simulink model "WK_MaoBi_Record"  (Simulink 7.7)
settings: Solver=ode4  StartTime=0.0  StopTime=inf  FixedStep=sample_time  RelTol=1e-3
InitFcn:
  | sample_time=0.005;%0.004;%0.0025;%0.02;
  | DeltaT = 0.02;
  | g = 9.81;
  | H0 = g%0.3165;
  | Kl = 1;
  | 
  | Omega_r = 1.6;%for Horizontal reference
  | Zeta_r = 0.7; %for Horizontal reference
  | Omega = 1.8;%for Horizontal Control
  | Zeta = 0.5;    %for Horizontal Control
  | 
  | Omega_h_r = 2.5; %for vertical reference
  | Zeta_h_r = 0.8;  %for vertical reference
  | Omega_h = 2.7;    %for vertical control
  | Zeta_h = 0.8;         %for vertical control
  | PI=pi;
  | 
  | Mass = 1;
  | Acc_Max = 4;
  | Acc_Max_h = 4;
  | 
  | Max_RP = 60;
undefined symbols (not defined in the file or in its folder): DiscIntNeverNeededParam
libraries: simulink x7, dspadpt3 x3, X330_Control x2, X400_Control x1
(part 1 of 2)
settings Model: Creator=ttcl3  LastModifiedBy=Vicon
settings SolverCC: MaxConsecutiveMinStep=auto
settings DebuggingCC: MultiTaskRateTransMsg=warning
settings SFSimCC: SimParseCustomCode=off

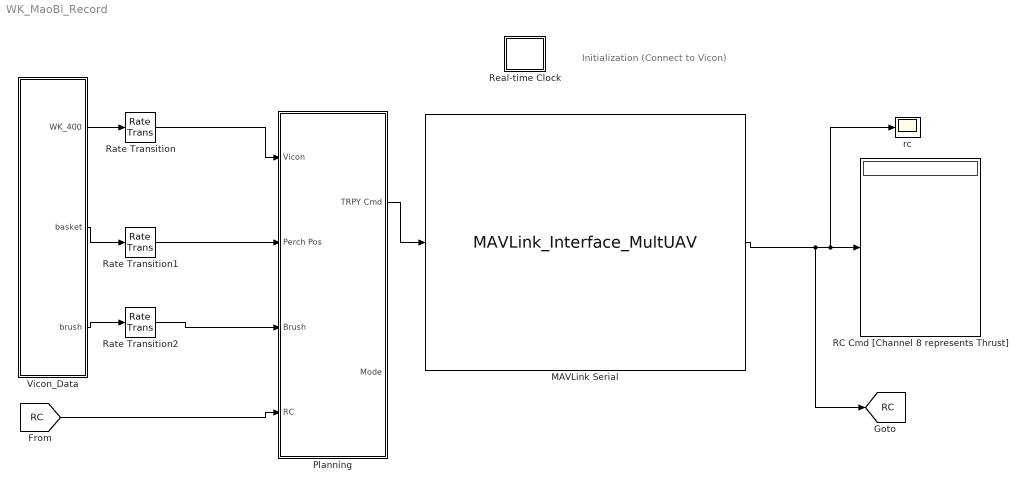
== system WK_MaoBi_Record ==
  note: Initialization
      | (Connect to Vicon)
  MAVLink Serial : S-Function  FunctionName=MAVLink_Interface_MultUAV  Parameters=COM_Port,Baud_Rate,MSG_INPUT,MSG_OUTPUT  EnableBusSupport=off  mask{COM_Port='COM8', Baud_Rate=57600, RC_SCALED=on, Quad_1=on, Quad_2=off, Quad_3=off}
      mask prompts: COM_Port "COM Port"; Baud_Rate "Baud Rate"; RC_SCALED "RC CHANNELS SCALED"; Quad_1 "Quad No 1"; Quad_2 "Quad No 2"; Quad_3 "Quad No 3"
      mask init:
      | MSG_ID_NUM_INPUT = [uint8(196) uint8(197) uint8(198)];
      | MSG_ID_NAME_INPUT = [Quad_1 Quad_2 Quad_3];
      | 
      | MSG_ID_NUM_OUTPUT = [uint8(34)];
      | MSG_ID_NAME_OUTPUT = [RC_SCALED];
      | 
      | idx_input = find(MSG_ID_NAME_INPUT);
      | MSG_INPUT = MSG_ID_NUM_INPUT(idx_input);
      | 
      | idx_output = find(MSG_ID_NAME_OUTPUT);
      | MSG_OUTPUT = MSG_ID_NUM_OUTPUT(idx_output);
      mask TabNameString: Setting,Setting,Output Message,Input Message,Input Message,Input Message
      mask Display:
      | % Block image
      | image(imread('10-inch Quad Heat Map.png'));
      | 
      | %Label block
      | fprintf('MAVLink Serial\n%s\n%dbps', COM_Port,  Baud_Rate)
      | 
      | 
      | %Label input ports
      | 
      | in = 1;
      | if (Quad_1 == 1)
      |     port_label('input', in, 'Quad 1');
      |     in = in + 1;
      | end
      | if (Quad_2 == 1)
      |     port_label('input', in, 'Quad 2');
      |     in = in + 1;
      | end
      | 
      | if (Quad_3 == 1)
      |     port_label('input', in, 'Quad 3');
      |     in = in + 1;
      | end
      | 
      | %Label output ports
      | 
      | out = 1;
      | if (RC_SCALED == 1)
      |     port_label('output', out, 'RC CMD');
      |     out = out + 1;
      | end
  Planning : Subsystem
  RC Cmd [Channel 8 represents Thrust] : Display
  Rate Transition : RateTransition  OutPortSampleTime=0.02
  Rate Transition1 : RateTransition  OutPortSampleTime=0.02
  Rate Transition2 : RateTransition  OutPortSampleTime=0.02
  Real-time Clock : Subsystem  mask(Real-time Clock){sample_time=0.02, tolerance=1}
      mask prompts: sample_time "Synchronize with real-time every n seconds:"; tolerance "Real-time warning tolerance (seconds):"
      mask help: Real-time Synchronization Block
      mask Help: This block synchronizes simulation time with the PC real-time clock or UNIX system clock. The first dialog entry is the period at which the clock is checked to insure real-time synchronization. The second dialog entry is the number of seconds that the simulation time must be within real-time before a warning is printed.
      mask Display: plot(0,0,100,100,[40,60,60,54,54,64,69,76,82,77,81,83,83,81,78,74,70,64,57,49,41,35,32,30,30,31,34,40,47,47,40,40],[90,90,85,85,80,79,76,87,80,70,64,57,49,41,33,28,24,22,21,23,25,31,37,46,56,65,73,78,80,85,85,90],[69,53,53],[64,50,73])
  Vicon_Data : Subsystem
  rc : Scope
      settings: TimeRange=10  YMin=-1  YMax=0.1
  tag scope: RC=global
  wires:
  [RC] -> Planning/4(RC)
  Planning/1(TRPY Cmd) -> MAVLink Serial/1
  MAVLink Serial/1 -> [RC], RC Cmd [Channel 8 represents Thrust]/1, rc/1
  Vicon_Data/1(WK_400) -> Rate Transition/1
  Vicon_Data/2(basket) -> Rate Transition1/1
  Rate Transition/1 -> Planning/1(Vicon)
  Rate Transition1/1 -> Planning/2(Perch Pos)
  Vicon_Data/3(brush) -> Rate Transition2/1
  Rate Transition2/1 -> Planning/3(Brush)

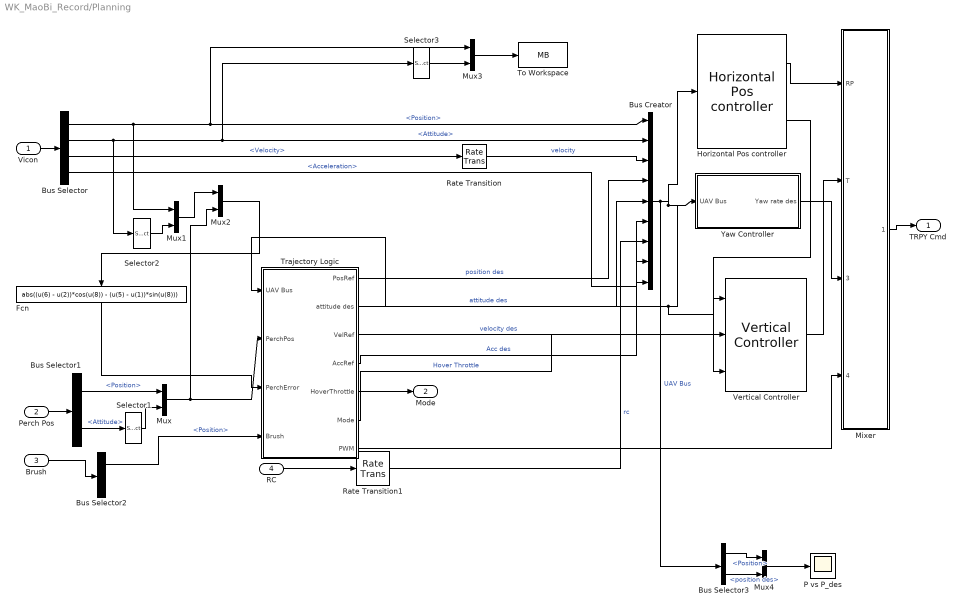
== system WK_MaoBi_Record/Planning ==
  Vicon : Inport
  Perch Pos : Inport  Port=2
  Brush : Inport  Port=3
  RC : Inport  Port=4
  Bus Creator : BusCreator  Inputs=9
  Bus Selector : BusSelector  OutputSignals=Position,Attitude,Velocity,Acceleration
  Bus Selector1 : BusSelector  OutputSignals=Position,Attitude
  Bus Selector2 : BusSelector  OutputSignals=Position,Attitude
  Bus Selector3 : BusSelector  OutputSignals=Position,position des
  Fcn : Fcn  Expr=abs((u(6) - u(2))*cos(u(8)) - (u(5) - u(1))*sin(u(8)))
  Horizontal Pos controller : X330_Control/Horizontal Pos controller  SystemSampleTime=-1  Max_RP=Max_RP  Omega=Omega  PID_i=1  Zeta=Zeta
  Mixer : Subsystem
  Mux{,1..4} (5 alike) : Mux  Inputs=2
  P vs P_des : Scope
      settings: YMin=-1.1  YMax=0.5
  Rate Transition : RateTransition  OutPortSampleTime=0.02
  Rate Transition1 : RateTransition  OutPortSampleTime=0.02
  Selector1 : Selector  InputPortWidth=3  IndexOptions=Index vector (dialog)  Indices=[3]  OutputSizes=1
  Selector2 : Selector  InputPortWidth=3  IndexOptions=Index vector (dialog)  Indices=[3]  OutputSizes=1
  Selector3 : Selector  InputPortWidth=3  IndexOptions=Index vector (dialog)  Indices=[3]  OutputSizes=1
  To Workspace : ToWorkspace  VariableName=MB  SampleTime=0.02  SaveFormat=Structure With Time
  Trajectory Logic : Subsystem
  Vertical Controller : X400_Control/Vertical Controller  SystemSampleTime=-1  Omega_h=Omega_h  Zeta_h=Zeta_h  PID_I_h=1  mass=Mass
  Yaw Controller : Subsystem
  TRPY Cmd : Outport
  Mode : Outport  Port=2
  wires:
  Horizontal Pos controller/1 -> Mixer/1(RP)
  Rate Transition/1 -> Bus Creator/3  "velocity"
  Rate Transition1/1 -> Bus Creator/7  "rc"
  Bus Creator/1 -> Yaw Controller/1(UAV Bus), Trajectory Logic/1(UAV Bus), Vertical Controller/1, Horizontal Pos controller/1, Bus Selector3/1  "UAV Bus"
  Yaw Controller/1(Yaw rate des) -> Mixer/3(Yaw rate)
  Vertical Controller/1 -> Mixer/2(T)
  Bus Selector/4 -> Bus Creator/8  "<Acceleration>"
  Trajectory Logic/1(PosRef) -> Bus Creator/4  "position des"
  Trajectory Logic/2(attitude des) -> Bus Creator/5  "attitude des"
  Trajectory Logic/3(VelRef) -> Bus Creator/6  "velocity des"
  Trajectory Logic/5(HoverThrottle) -> Vertical Controller/2  "Hover Throttle"
  Bus Selector/1 -> Mux1/1, Bus Creator/1, Mux3/1  "<Position>"
  Bus Selector/2 -> Selector2/1, Bus Creator/2, Selector3/1  "<Attitude>"
  Bus Selector/3 -> Rate Transition/1  "<Velocity>"
  Vicon/1 -> Bus Selector/1
  Mixer/1(XYZ RPY) -> TRPY Cmd/1
  Trajectory Logic/4(AccRef) -> Bus Creator/9  "Acc des"
  Mux/1 -> Trajectory Logic/2(PerchPos), Mux2/2
  Trajectory Logic/6(Mode) -> Mode/1
  RC/1 -> Rate Transition1/1
  Trajectory Logic/7(PWM) -> Mixer/4(PWM)
  Perch Pos/1 -> Bus Selector1/1
  Bus Selector1/1 -> Mux/1  "<Position>"
  Bus Selector1/2 -> Selector1/1  "<Attitude>"
  Selector1/1 -> Mux/2
  Selector2/1 -> Mux1/2
  Mux2/1 -> Fcn/1
  Mux1/1 -> Mux2/1
  Fcn/1 -> Trajectory Logic/3(PerchError)
  Horizontal Pos controller/2 -> Vertical Controller/3
  Brush/1 -> Bus Selector2/1
  Bus Selector2/1 -> Trajectory Logic/4(Brush)  "<Position>"
  Mux3/1 -> To Workspace/1
  Selector3/1 -> Mux3/2
  Mux4/1 -> P vs P_des/1
  Bus Selector3/1 -> Mux4/1  "<Position>"
  Bus Selector3/2 -> Mux4/2  "<position des>"

== system WK_MaoBi_Record/Real-time Clock ==
  Real-time Clock : S-Function  FunctionName=rtclock  Parameters=sample_time, tolerance  EnableBusSupport=off

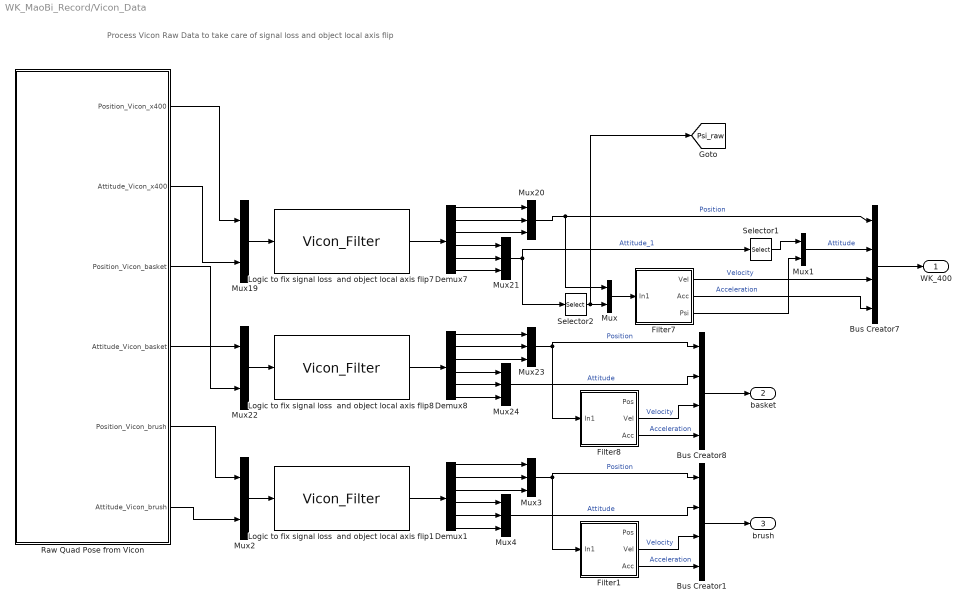
== system WK_MaoBi_Record/Vicon_Data ==
  note: Process Vicon Raw Data to take care of signal loss and object local axis flip
  Bus Creator1 : BusCreator
  Bus Creator7 : BusCreator
  Bus Creator8 : BusCreator
  Demux1 : Demux  Outputs=6
  Demux7 : Demux  Outputs=6
  Demux8 : Demux  Outputs=6
  Filter1 : Subsystem
  Filter7 : Subsystem
  Filter8 : Subsystem
  Logic to fix signal loss  and object local axis flip1 : M-S-Function  FunctionName=Vicon_Filter
  Logic to fix signal loss  and object local axis flip7 : M-S-Function  FunctionName=Vicon_Filter
  Logic to fix signal loss  and object local axis flip8 : M-S-Function  FunctionName=Vicon_Filter
  Mux{,1..2,19,22} (5 alike) : Mux  Inputs=2
  Mux{3..4,20..21,23..24} (6 alike) : Mux  Inputs=3
  Raw Quad Pose from Vicon : Subsystem
  Selector1 : Selector  InputPortWidth=3  IndexOptions=Index vector (dialog)  Indices=[1 2]  OutputSizes=1
  Selector2 : Selector  InputPortWidth=3  IndexOptions=Index vector (dialog)  Indices=[3]  OutputSizes=1
  WK_400 : Outport
  basket : Outport  Port=2
  brush : Outport  Port=3
  tag scope: Psi_raw=global
  wires:
  Mux19/1 -> Logic to fix signal loss  and object local axis flip7/1
  Logic to fix signal loss  and object local axis flip7/1 -> Demux7/1
  Demux7/3 -> Mux20/3
  Demux7/4 -> Mux21/1
  Demux7/5 -> Mux21/2
  Demux7/6 -> Mux21/3
  Bus Creator7/1 -> WK_400/1
  Demux7/1 -> Mux20/1
  Demux7/2 -> Mux20/2
  Mux20/1 -> Bus Creator7/1, Mux/1  "Position"
  Mux22/1 -> Logic to fix signal loss  and object local axis flip8/1
  Logic to fix signal loss  and object local axis flip8/1 -> Demux8/1
  Demux8/3 -> Mux23/3
  Demux8/4 -> Mux24/1
  Demux8/5 -> Mux24/2
  Demux8/6 -> Mux24/3
  Filter8/2(Vel) -> Bus Creator8/3  "Velocity"
  Filter8/3(Acc) -> Bus Creator8/4  "Acceleration"
  Mux24/1 -> Bus Creator8/2  "Attitude"
  Bus Creator8/1 -> basket/1
  Demux8/1 -> Mux23/1
  Demux8/2 -> Mux23/2
  Mux23/1 -> Filter8/1(In1), Bus Creator8/1  "Position"
  Raw Quad Pose from Vicon/1(Position_Vicon_x400) -> Mux19/1
  Raw Quad Pose from Vicon/2(Attitude_Vicon_x400) -> Mux19/2
  Raw Quad Pose from Vicon/3(Position_Vicon_basket) -> Mux22/1
  Raw Quad Pose from Vicon/4(Attitude_Vicon_basket) -> Mux22/2
  Mux21/1 -> Selector2/1, Selector1/1  "Attitude_1"
  Filter7/1(Vel) -> Bus Creator7/3  "Velocity"
  Filter7/2(Acc) -> Bus Creator7/4  "Acceleration"
  Selector2/1 -> Mux/2, [Psi_raw]
  Mux/1 -> Filter7/1(In1)
  Filter7/3(Psi) -> Mux1/2
  Selector1/1 -> Mux1/1
  Mux1/1 -> Bus Creator7/2  "Attitude"
  Mux2/1 -> Logic to fix signal loss  and object local axis flip1/1
  Logic to fix signal loss  and object local axis flip1/1 -> Demux1/1
  Demux1/3 -> Mux3/3
  Demux1/4 -> Mux4/1
  Demux1/5 -> Mux4/2
  Demux1/6 -> Mux4/3
  Filter1/2(Vel) -> Bus Creator1/3  "Velocity"
  Filter1/3(Acc) -> Bus Creator1/4  "Acceleration"
  Mux4/1 -> Bus Creator1/2  "Attitude"
  Bus Creator1/1 -> brush/1
  Demux1/1 -> Mux3/1
  Demux1/2 -> Mux3/2
  Mux3/1 -> Bus Creator1/1, Filter1/1(In1)  "Position"
  Raw Quad Pose from Vicon/5(Position_Vicon_brush) -> Mux2/1
  Raw Quad Pose from Vicon/6(Attitude_Vicon_brush) -> Mux2/2

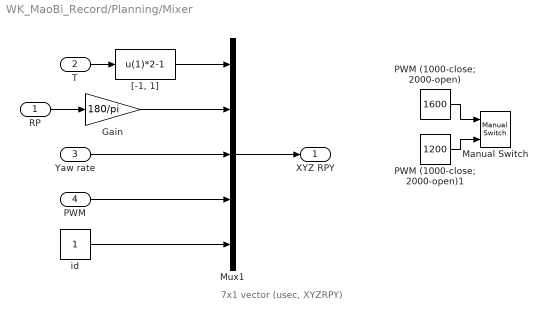
== system WK_MaoBi_Record/Planning/Mixer ==
  note: 7x1 vector (usec, XYZRPY)
  RP : Inport
  T : Inport  Port=2
  Yaw rate : Inport  Port=3
  PWM : Inport  Port=4
  Gain : Gain  Gain=180/pi
  Manual Switch : simulink/Signal Routing/Manual Switch  SystemSampleTime=-1  sw=1  action=0  varsize=off
  Mux1 : Mux  Inputs=5
  PWM (1000-close; 2000-open) : Constant  Value=1600  SampleTime=0.02
  PWM (1000-close; 2000-open)1 : Constant  Value=1200  SampleTime=0.02
  "[-1, 1]" : Fcn  Expr=u(1)*2-1
  id : Constant  SampleTime=0.02
  XYZ RPY : Outport
  wires:
  Mux1/1 -> XYZ RPY/1
  T/1 -> "[-1, 1]"/1
  RP/1 -> Gain/1
  Yaw rate/1 -> Mux1/3
  id/1 -> Mux1/5
  PWM (1000-close; 2000-open)/1 -> Manual Switch/1
  PWM (1000-close; 2000-open)1/1 -> Manual Switch/2
  PWM/1 -> Mux1/4
  Gain/1 -> Mux1/2
  "[-1, 1]"/1 -> Mux1/1

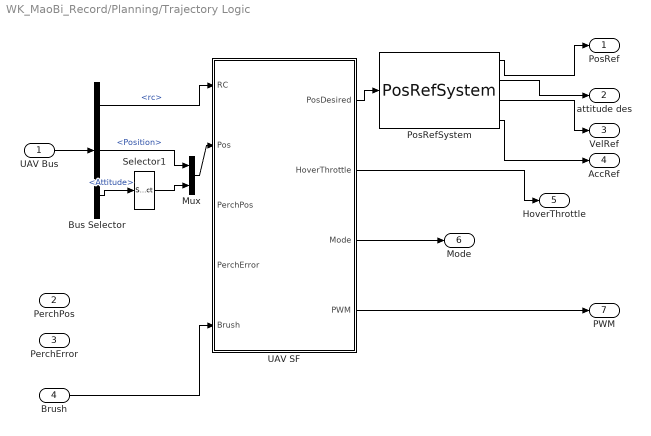
== system WK_MaoBi_Record/Planning/Trajectory Logic ==
  UAV Bus : Inport
  PerchPos : Inport  Port=2
  PerchError : Inport  Port=3
  Brush : Inport  Port=4
  Bus Selector : BusSelector  OutputSignals=rc,Position,Attitude
  Mux : Mux  Inputs=2
  PosRefSystem : X330_Control/PosRefSystem  SystemSampleTime=-1  Omega_r=Omega_r  Zeta_r=Zeta_r  Acc_Max=Acc_Max  Omega_h_r=Omega_h_r  Zeta_h_r=Zeta_h_r  Acc_h_Max=Acc_Max_h
  Selector1 : Selector  InputPortWidth=3  IndexOptions=Index vector (dialog)  Indices=[3]  OutputSizes=1
  UAV SF : Stateflow chart  TreatAsAtomicUnit=on
  PosRef : Outport
  attitude des : Outport  Port=2
  VelRef : Outport  Port=3
  AccRef : Outport  Port=4
  HoverThrottle : Outport  Port=5
  Mode : Outport  Port=6
  PWM : Outport  Port=7
  wires:
  UAV SF/1(PosDesired) -> PosRefSystem/1
  Bus Selector/1 -> UAV SF/1(RC)  "<rc>"
  UAV SF/2(HoverThrottle) -> HoverThrottle/1
  UAV SF/3(Mode) -> Mode/1
  UAV Bus/1 -> Bus Selector/1
  Bus Selector/2 -> Mux/1  "<Position>"
  Bus Selector/3 -> Selector1/1  "<Attitude>"
  Selector1/1 -> Mux/2
  Mux/1 -> UAV SF/2(Pos)
  UAV SF/4(PWM) -> PWM/1
  PosRefSystem/1 -> PosRef/1
  PosRefSystem/3 -> VelRef/1
  PosRefSystem/4 -> AccRef/1
  PosRefSystem/2 -> attitude des/1
  Brush/1 -> UAV SF/5(Brush)

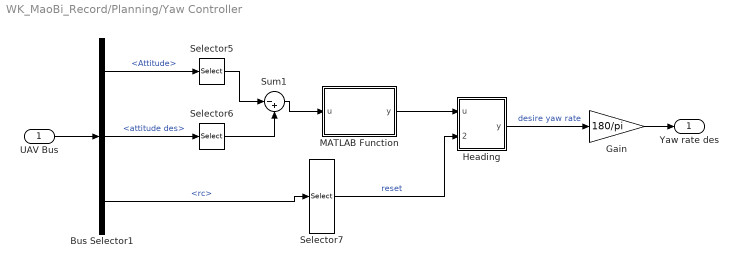
== system WK_MaoBi_Record/Planning/Yaw Controller ==
  UAV Bus : Inport
  Bus Selector1 : BusSelector  OutputSignals=Attitude,attitude des,rc
  Gain : Gain  Gain=180/pi
  Heading : Subsystem  AncestorBlock=simulink/Continuous/PID Controller  DialogController=pidpack.PIDConfig.pidDDGCreate  DialogControllerArgs=DataTag0  mask(PID 1dof){Controller=PI, TimeDomain=Discrete-time, SampleTime=0.02, IntegratorMethod=Trapezoidal, FilterMethod=Trapezoidal, Form=Parallel, P=3, I=1, D=0, N=100, InitialConditionSource=internal, InitialConditionForIntegrator=0, InitialConditionForFilter=0, ExternalReset=rising, IgnoreLimit=off, ZeroCross=on, LimitOutput=on, UpperSaturationLimit=300*pi/180, LowerSaturationLimit=-300*pi/180, LinearizeAsGain=off, AntiWindupMode=none, Kb=1, TrackingMode=off, Kt=1, RndMeth=Floor, SaturateOnIntegerOverflow=off, LockScale=off, PParamMin=[], PParamMax=[], PParamDataTypeStr=Inherit: Inherit via internal rule, IParamMin=[], IParamMax=[], IParamDataTypeStr=Inherit: Inherit via internal rule, DParamMin=[], DParamMax=[], DParamDataTypeStr=Inherit: Inherit via internal rule, NParamMin=[], NParamMax=[], NParamDataTypeStr=Inherit: Inherit via internal rule, KbParamMin=[], KbParamMax=[], KbParamDataTypeStr=Inherit: Inherit via internal rule, KtParamMin=[], KtParamMax=[], KtParamDataTypeStr=Inherit: Inherit via internal rule, POutMin=[], POutMax=[], POutDataTypeStr=Inherit: Inherit via internal rule, IOutMin=[], IOutMax=[], IOutDataTypeStr=Inherit: Inherit via internal rule, DOutMin=[], DOutMax=[], DOutDataTypeStr=Inherit: Inherit via internal rule, NOutMin=[], NOutMax=[], NOutDataTypeStr=Inherit: Inherit via internal rule, KbOutMin=[], KbOutMax=[], KbOutDataTypeStr=Inherit: Inherit via internal rule, KtOutMin=[], KtOutMax=[], KtOutDataTypeStr=Inherit: Inherit via internal rule, IntegratorOutMin=[], IntegratorOutMax=[], IntegratorOutDataTypeStr=Inherit: Inherit via internal rule, FilterOutMin=[], FilterOutMax=[], FilterOutDataTypeStr=Inherit: Inherit via internal rule, SumOutMin=[], SumOutMax=[], SumOutDataTypeStr=Inherit: Inherit via internal rule, SumI1OutMin=[], SumI1OutMax=[], SumI1OutDataTypeStr=Inherit: Inherit via internal rule, SumI2OutMin=[], SumI2OutMax=[], SumI2OutDataTypeStr=Inherit: Inherit via internal rule, SumI3OutMin=[], SumI3OutMax=[], SumI3OutDataTypeStr=Inherit: Inherit via internal rule, SumDOutMin=[], SumDOutMax=[], SumDOutDataTypeStr=Inherit: Inherit via internal rule, SumAccumDataTypeStr=Inherit: Inherit via internal rule, SumI1AccumDataTypeStr=Inherit: Inherit via internal rule, SumI2AccumDataTypeStr=Inherit: Inherit via internal rule, SumI3AccumDataTypeStr=Inherit: Inherit via internal rule, SumDAccumDataTypeStr=Inherit: Inherit via internal rule, SaturationOutMin=[], SaturationOutMax=[], SaturationOutDataTypeStr=Inherit: Same as input, IntegratorContinuousStateAttributes='', IntegratorStateIdentifier=, IntegratorStateMustResolveToSignalObject=off, IntegratorRTWStateStorageClass=Auto, IntegratorRTWStateStorageTypeQualifier=, FilterContinuousStateAttributes='', FilterStateIdentifier=, FilterStateMustResolveToSignalObject=off, FilterRTWStateStorageClass=Auto, FilterRTWStateStorageTypeQualifier=}
      mask prompts: TimeDomain "Time domain:"; SampleTime "Sample time (-1 for inherited):"; IntegratorMethod "Integrator method:"; FilterMethod "Filter method:"; P "Proportional (P):"; I "Integral (I):"; D "Derivative (D):"; N "Filter coefficient (N):"; InitialConditionSource "Source:"; InitialConditionForIntegrator "Integrator:"; InitialConditionForFilter "Filter:"; ExternalReset "External reset:"; IgnoreLimit "Ignore reset when linearizing"; ZeroCross "Enable zero-crossing detection"; LimitOutput "Limit output"; UpperSaturationLimit "Upper saturation limit:"; LowerSaturationLimit "Lower saturation limit:"; LinearizeAsGain "Ignore saturation when linearizing"; AntiWindupMode "Anti-windup method:"; Kb "Back-calculation coefficient (Kb):"; TrackingMode "Enable tracking mode"; Kt "Tracking coefficient (Kt):"; RndMeth "Integer rounding mode:"; SaturateOnIntegerOverflow "Saturate on integer overflow"; LockScale "Lock data type settings against changes by the fixed-point tools"; PParamMin "P parameter minimum:"; PParamMax "P parameter maximum:"; PParamDataTypeStr "P parameter:"; IParamMin "I parameter minimum:"; IParamMax "I parameter maximum:"; IParamDataTypeStr "I parameter:"; DParamMin "D parameter minimum:"; DParamMax "D parameter maximum:"; DParamDataTypeStr "D parameter:"; NParamMin "N parameter minimum:"; NParamMax "N parameter maximum:"; NParamDataTypeStr "N parameter:"; KbParamMin "Kb parameter minimum:"; KbParamMax "Kb parameter maximum:"; KbParamDataTypeStr "Kb parameter:"; KtParamMin "Kt parameter minimum:"; KtParamMax "Kt parameter maximum:"; KtParamDataTypeStr "Kt parameter:"; POutMin "P product output minimum:"; POutMax "P product output maximum:"; POutDataTypeStr "P product output:"; IOutMin "I product output minimum:"; IOutMax "I product output maximum:"; IOutDataTypeStr "I product output:"; DOutMin "D product output minimum:"; DOutMax "D product output maximum:"; DOutDataTypeStr "D product output:"; NOutMin "N product output minimum:"; NOutMax "N product output maximum:"; NOutDataTypeStr "N product output:"; KbOutMin "Kb product output minimum:"; KbOutMax "Kb product output maximum:"; KbOutDataTypeStr "Kb product output:"; KtOutMin "Kt product output minimum:"; KtOutMax "Kt product output maximum:"; KtOutDataTypeStr "Kt product output:"; IntegratorOutMin "Integrator output minimum:"; IntegratorOutMax "Integrator output maximum:"; IntegratorOutDataTypeStr "Integrator output:"; FilterOutMin "Filter output minimum:"; FilterOutMax "Filter output maximum:"; FilterOutDataTypeStr "Filter output:"; SumOutMin "Sum output minimum:"; SumOutMax "Sum output maximum:"; SumOutDataTypeStr "Sum output:"; SumI1OutMin "SumI1 output minimum:"; SumI1OutMax "SumI1 output maximum:"; SumI1OutDataTypeStr "SumI1 output:"; SumI2OutMin "SumI2 output minimum:"; SumI2OutMax "SumI2 output maximum:"; SumI2OutDataTypeStr "SumI2 output:"; SumI3OutMin "SumI3 output minimum:"; SumI3OutMax "SumI3 output maximum:"; SumI3OutDataTypeStr "SumI3 output:"; SumDOutMin "SumD output minimum:"; SumDOutMax "SumD output maximum:"; SumDOutDataTypeStr "SumD output:"; SumAccumDataTypeStr "Accumulator of Sum:"; SumI1AccumDataTypeStr "Accumulator of SumI1:"; SumI2AccumDataTypeStr "Accumulator of SumI2:"; SumI3AccumDataTypeStr "Accumulator of SumI3:"; SumDAccumDataTypeStr "Accumulator of SumD:"; SaturationOutMin "Saturation output minimum:"; SaturationOutMax "Saturation output maximum:"; SaturationOutDataTypeStr "Saturation output:"; IntegratorContinuousStateAttributes "State name: (e.g., 'position')"; IntegratorStateIdentifier "State name:"; IntegratorStateMustResolveToSignalObject "State name must resolve to Simulink signal object"; IntegratorRTWStateStorageClass "Code generation storage class:"; IntegratorRTWStateStorageTypeQualifier "Code generation storage type qualifier:"; FilterContinuousStateAttributes "State name: (e.g., 'position')"; FilterStateIdentifier "State name:"; FilterStateMustResolveToSignalObject "State name must resolve to Simulink signal object"; FilterRTWStateStorageClass "Code generation storage class:"; FilterRTWStateStorageTypeQualifier "Code generation storage type qualifier:"
      mask help: This block implements continuous- and discrete-time PID control algorithms and includes advanced features such as anti-windup, external reset, and signal tracking. You can tune the PID gains automatically using the 'Tune...' button (requires Simulink Control Design).
      mask init:
      | pidpack.PIDConfig.configPID(gcbh);
      settings: DeleteFcn=pidpack.PIDConfig.closeTuner(gcbh)  ModelCloseFcn=pidpack.PIDConfig.closeTuner(gcbh)  NameChangeFcn=pidpack.PIDConfig.updateTunerName(gcbh)
      mask StyleString: popup(PID|PI|PD|P|I),popup(Continuous-time|Discrete-time),edit,popup(Forward Euler|Backward Euler|Trapezoidal),popup(Forward Euler|Backward Euler|Trapezoidal),popup(Ideal|Parallel),edit,edit,edit,edit,popup(internal|external),edit,edit,popup(none|rising|falling|either|level),checkbox,checkbox,checkbox,edit,edit,checkbox,popup(none|back-calculation|clamping),edit,checkbox,edit,popup(Ceiling|Convergent|Floor|Nearest|Round|Simplest|Zero),checkbox,checkbox,min,max,unidt({a=30|28|29|}{i=Inherit: Inherit via internal rule|Inherit: Same as input}{b=double|single|int8|uint8|int16|uint16|int32|uint32}{s=UDTBinaryPointMode|UDTSlopeBiasMode|UDTBestPrecisionMode}{g=UDTSignedSign|UDTUnsignedSign}),min,max,unidt({a=33|31|32|}{i=Inherit: Inherit via internal rule|Inherit: Same as input}{b=double|single|int8|uint8|int16|uint16|int32|uint32}{s=UDTBinaryPointMode|UDTSlopeBiasMode|UDTBestPrecisionMode}{g=UDTSignedSign|UDTUnsignedSign}),min,max,unidt({a=36|34|35|}{i=Inherit: Inherit via internal rule|Inherit: Same as input}{b=double|single|int8|uint8|int16|uint16|int32|uint32}{s=UDTBinaryPointMode|UDTSlopeBiasMode|UDTBestPrecisionMode}{g=UDTSignedSign|UDTUnsignedSign}),min,max,unidt({a=39|37|38|}{i=Inherit: Inherit via internal rule|Inherit: Same as input}{b=double|single|int8|uint8|int16|uint16|int32|uint32}{s=UDTBinaryPointMode|UDTSlopeBiasMode|UDTBestPrecisionMode}{g=UDTSignedSign|UDTUnsignedSign}),min,max,unidt({a=42|40|41|}{i=Inherit: Inherit via internal rule|Inherit: Same as input}{b=double|single|int8|uint8|int16|uint16|int32|uint32}{s=UDTBinaryPointMode|UDTSlopeBiasMode|UDTBestPrecisionMode}{g=UDTSignedSign|UDTUnsignedSign}),min,max,unidt({a=45|43|44|}{i=Inherit: Inherit via internal rule|Inherit: Same as input}{b=double|single|int8|uint8|int16|uint16|int32|uint32}{s=UDTBinaryPointMode|UDTSlopeBiasMode|UDTBestPrecisionMode}{g=UDTSignedSign|UDTUnsignedSign}),min,max,unidt({a=48|46|47|}{i=Inherit: Inherit via internal rule|Inherit: Inherit via back propagation|Inherit: Same as input}{b=double|single|int8|uint8|int16|uint16|int32|uint32}{s=UDTBinaryPointMode|UDTSlopeBiasMode}{g=UDTSignedSign|UDTUnsignedSign}),min,max,unidt({a=51|49|50|}{i=Inherit: Inherit via internal rule|Inherit: Inherit via back propagation|Inherit: Same as input}{b=double|single|int8|uint8|int16|uint16|int32|uint32}{s=UDTBinaryPointMode|UDTSlopeBiasMode}{g=UDTSignedSign|UDTUnsignedSign}),min,max,unidt({a=54|52|53|}{i=Inherit: Inherit via internal rule|Inherit: Inherit via back propagation|Inherit: Same as input}{b=double|single|int8|uint8|int16|uint16|int32|uint32}{s=UDTBinaryPointMode|UDTSlopeBiasMode}{g=UDTSignedSign|UDTUnsignedSign}),min,max,unidt({a=57|55|56|}{i=Inherit: Inherit via internal rule|Inherit: Inherit via back propagation|Inherit: Same as input}{b=double|single|int8|uint8|int16|uint16|int32|uint32}{s=UDTBinaryPointMode|UDTSlopeBiasMode}{g=UDTSignedSign|UDTUnsignedSign}),min,max,unidt({a=60|58|59|}{i=Inherit: Inherit via internal rule|Inherit: Inherit via back propagation|Inherit: Same as input}{b=double|single|int8|uint8|int16|uint16|int32|uint32}{s=UDTBinaryPointMode|UDTSlopeBiasMode}{g=UDTSignedSign|UDTUnsignedSign}),min,max,unidt({a=63|61|62|}{i=Inherit: Inherit via internal rule|Inherit: Inherit via back propagation|Inherit: Same as input}{b=double|single|int8|uint8|int16|uint16|int32|uint32}{s=UDTBinaryPointMode|UDTSlopeBiasMode}{g=UDTSignedSign|UDTUnsignedSign}),min,max,unidt({a=66|64|65|}{i=Inherit: Inherit via internal rule|Inherit: Inherit via back propagation}{b=double|single|int8|uint8|int16|uint16|int32|uint32}{s=UDTBinaryPointMode|UDTSlopeBiasMode}{g=UDTSignedSign|UDTUnsignedSign}),min,max,unidt({a=69|67|68|}{i=Inherit: Inherit via internal rule|Inherit: Inherit via back propagation}{b=double|single|int8|uint8|int16|uint16|int32|uint32}{s=UDTBinaryPointMode|UDTSlopeBiasMode}{g=UDTSignedSign|UDTUnsignedSign}),min,max,unidt({a=72|70|71|}{i=Inherit: Inherit via internal rule|Inherit: Inherit via back propagation|Inherit: Same as first input|Inherit: Same as accumulator}{b=double|single|int8|uint8|int16|uint16|int32|uint32}{s=UDTBinaryPointMode|UDTSlopeBiasMode}{g=UDTSignedSign|UDTUnsignedSign}),min,max,unidt({a=75|73|74|}{i=Inherit: Inherit via internal rule|Inherit: Inherit via back propagation|Inherit: Same as first input|Inherit: Same as accumulator}{b=double|single|int8|uint8|int16|uint16|int32|uint32}{s=UDTBinaryPointMode|UDTSlopeBiasMode}{g=UDTSignedSign|UDTUnsignedSign}),min,max,unidt({a=78|76|77|}{i=Inherit: Inherit via internal rule|Inherit: Inherit via back propagation|Inherit: Same as first input|Inherit: Same as accumulator}{b=double|single|int8|uint8|int16|uint16|int32|uint32}{s=UDTBinaryPointMode|UDTSlopeBiasMode}{g=UDTSignedSign|UDTUnsignedSign}),min,max,unidt({a=81|79|80|}{i=Inherit: Inherit via internal rule|Inherit: Inherit via back propagation|Inherit: Same as first input|Inherit: Same as accumulator}{b=double|single|int8|uint8|int16|uint16|int32|uint32}{s=UDTBinaryPointMode|UDTSlopeBiasMode}{g=UDTSignedSign|UDTUnsignedSign}),min,max,unidt({a=84|82|83|}{i=Inherit: Inherit via internal rule|Inherit: Inherit via back propagation|Inherit: Same as first input|Inherit: Same as accumulator}{b=double|single|int8|uint8|int16|uint16|int32|uint32}{s=UDTBinaryPointMode|UDTSlopeBiasMode}{g=UDTSignedSign|UDTUnsignedSign}),unidt({a=85|||}{i=Inherit: Inherit via internal rule|Inherit: Same as first input}{b=double|single|int8|uint8|int16|uint16|int32|uint32}{s=UDTBinaryPointMode|UDTSlopeBiasMode}{g=UDTSignedSign|UDTUnsignedSign}),unidt({a=86|||}{i=Inherit: Inherit via internal rule|Inherit: Same as first input}{b=double|single|int8|uint8|int16|uint16|int32|uint32}{s=UDTBinaryPointMode|UDTSlopeBiasMode}{g=UDTSignedSign|UDTUnsignedSign}),unidt({a=87|||}{i=Inherit: Inherit via internal rule|Inherit: Same as first input}{b=double|single|int8|uint8|int16|uint16|int32|uint32}{s=UDTBinaryPointMode|UDTSlopeBiasMode}{g=UDTSignedSign|UDTUnsignedSign}),unidt({a=88|||}{i=Inherit: Inherit via internal rule|Inherit: Same as first input}{b=double|single|int8|uint8|int16|uint16|int32|uint32}{s=UDTBinaryPointMode|UDTSlopeBiasMode}{g=UDTSignedSign|UDTUnsignedSign}),unidt({a=89|||}{i=Inherit: Inherit via internal rule|Inherit: Same as first input}{b=double|single|int8|uint8|int16|uint16|int32|uint32}{s=UDTBinaryPointMode|UDTSlopeBiasMode}{g=UDTSignedSign|UDTUnsignedSign}),min,max,unidt({a=92|90|91|}{i=Inherit: Inherit via back propagation|Inherit: Same as input}{b=double|single|int8|uint8|int16|uint16|int32|uint32}{s=UDTBinaryPointMode|UDTSlopeBiasMode}{g=UDTSignedSign|UDTUnsignedSign}),edit,edit,checkbox,popup(Auto|ExportedGlobal|ImportedExtern|ImportedExternPointer),edit,edit,edit,checkbox,popup(Auto|ExportedGlobal|ImportedExtern|ImportedExternPointer),edit
      mask Display:
      | disp('PI(z)')
      | port_label('input',1, '');
      | port_label('output',1, '');plot([0 4 4 7]+2,[0 0 8 8]+8);
      | plot([1 4 6]+2,[3 6 3]+8);
      | plot([0 4 6 10]+32,[0 0 8 8]+18);
  MATLAB Function : Stateflow chart  TreatAsAtomicUnit=on
  Selector5 : Selector  InputPortWidth=3  IndexOptions=Index vector (dialog)  Indices=[3]  OutputSizes=1
  Selector6 : Selector  InputPortWidth=3  IndexOptions=Index vector (dialog)  Indices=[3]  OutputSizes=1
  Selector7 : Selector  InputPortWidth=8  IndexOptions=Index vector (dialog)  Indices=[5]  OutputSizes=1
  Sum1 : Sum  Inputs=|-+
  Yaw rate des : Outport
  wires:
  Gain/1 -> Yaw rate des/1
  Selector5/1 -> Sum1/1
  Selector7/1 -> Heading/2(RESET)  "reset"
  Heading/1(y) -> Gain/1  "desire yaw rate"
  Bus Selector1/1 -> Selector5/1  "<Attitude>"
  UAV Bus/1 -> Bus Selector1/1
  MATLAB Function/1(y) -> Heading/1(u)
  Sum1/1 -> MATLAB Function/1(u)
  Selector6/1 -> Sum1/2
  Bus Selector1/2 -> Selector6/1  "<attitude des>"
  Bus Selector1/3 -> Selector7/1  "<rc>"

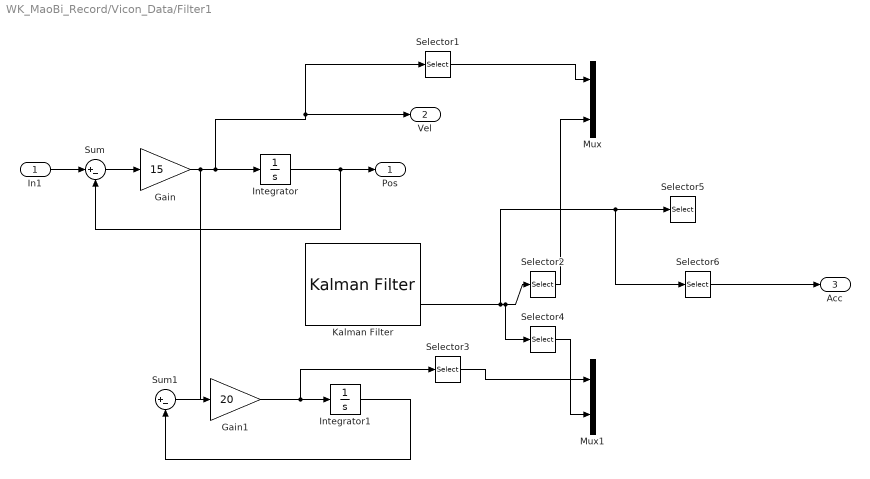
== system WK_MaoBi_Record/Vicon_Data/Filter1 ==
  In1 : Inport
  Gain : Gain  Gain=15
  Gain1 : Gain  Gain=20
  Integrator : Integrator
  Integrator1 : Integrator
  Kalman Filter : dspadpt3/Kalman Filter  SystemSampleTime=-1  num_targets=1  sourceEnable=Always  isReset=on  X=zeros([9, 1])  P=zeros(9)  A=[1 sample_time sample_time*sample_time/2 zeros(1,6);0 1 sample_time zeros(1,6);0 0 1 zeros(1,6);0 0 0 1 sample_time sample_time*sample_time/2 0 0 0;zeros(1,4) 1 sample_time zeros(1,3);zeros(1,5) 1 zeros(1,3);zeros(1,6) 1 sample_time sample_time*sample_time/2;zeros(1,7) 1 sample_time;zeros(1,8) 1]  sourceMeasure=Specify via Dialog  H=[1 zeros(1,8); zeros(1,3) 1 zeros(1,5);zeros(1,6) 1 0 0]  Q=diag([0 0.001 0.001 0 0.001 0.001 0 0.001 0.001])  R=0.001*eye(3)  isOutputEstMeasure=on  isOutputEstState=on  isOutputEstError=off  isOutputPrdMeasure=off  isOutputPrdState=off  isOutputPrdError=off
  Mux : Mux  Inputs=2
  Mux1 : Mux  Inputs=2
  Selector1 : Selector  InputPortWidth=3  IndexOptions=Index vector (dialog)  Indices=[2]  OutputSizes=1
  Selector2 : Selector  InputPortWidth=9  IndexOptions=Index vector (dialog)  Indices=[5]  OutputSizes=1
  Selector3 : Selector  InputPortWidth=3  IndexOptions=Index vector (dialog)  Indices=[2]  OutputSizes=1
  Selector4 : Selector  InputPortWidth=9  IndexOptions=Index vector (dialog)  Indices=[6]  OutputSizes=1
  Selector5 : Selector  InputPortWidth=9  IndexOptions=Index vector (dialog)  Indices=[2 5 8]  OutputSizes=1
  Selector6 : Selector  InputPortWidth=9  IndexOptions=Index vector (dialog)  Indices=[3 6 9]  OutputSizes=1
  Sum : Sum  Inputs=|+-
  Sum1 : Sum  Inputs=|+-
  Pos : Outport
  Vel : Outport  Port=2
  Acc : Outport  Port=3
  wires:
  Selector6/1 -> Acc/1
  Selector4/1 -> Mux1/2
  Selector3/1 -> Mux1/1
  Selector2/1 -> Mux/2
  Integrator1/1 -> Sum1/2
  Gain1/1 -> Selector3/1, Integrator1/1
  Sum1/1 -> Gain1/1
  Kalman Filter/2 -> Selector6/1, Selector5/1, Selector2/1, Selector4/1
  Selector1/1 -> Mux/1
  In1/1 -> Sum/1
  Integrator/1 -> Sum/2, Pos/1
  Gain/1 -> Sum1/1, Vel/1, Selector1/1, Integrator/1
  Sum/1 -> Gain/1

== system WK_MaoBi_Record/Vicon_Data/Filter7 ==
  In1 : Inport
  Kalman Filter : dspadpt3/Kalman Filter  SystemSampleTime=-1  num_targets=1  sourceEnable=Always  isReset=on  X=zeros([12, 1])  P=zeros(12)  A=[1 sample_time sample_time*sample_time/2 zeros(1,9);0 1 sample_time zeros(1,9);0 0 1 zeros(1,9);0 0 0 1 sample_time sample_time*sample_time/2 zeros(1,6);zeros(1,4) 1 sample_time zeros(1,6);zeros(1,5) 1 zeros(1,6);zeros(1,6) 1 sample_time sample_time*sample_time/2 zeros(1,3);zeros(1,7) 1 sample_time zeros(1,3);zeros(1,8) 1 zeros(1,3);zeros(1,9) 1 sample_time sample_time*sample_time/2;zeros(1,10) 1 sample_time;zeros(1,11) 1];  sourceMeasure=Specify via Dialog  H=[1 zeros(1,11); zeros(1,3) 1 zeros(1,8);zeros(1,6) 1 zeros(1,5);zeros(1,9) 1 0 0]  Q=diag([0 0.001 0.001 0 0.001 0.001 0 0.001 0.001 0 0.001 0.001]);  R=diag([0.001 0.001 0.001 0.05])  isOutputEstMeasure=off  isOutputEstState=on  isOutputEstError=off  isOutputPrdMeasure=off  isOutputPrdState=off  isOutputPrdError=off
  Selector1 : Selector  InputPortWidth=12  IndexOptions=Index vector (dialog)  Indices=[10]  OutputSizes=1
  Selector5 : Selector  InputPortWidth=12  IndexOptions=Index vector (dialog)  Indices=[2 5 8]  OutputSizes=1
  Selector6 : Selector  InputPortWidth=12  IndexOptions=Index vector (dialog)  Indices=[3 6 9]  OutputSizes=1
  Vel : Outport
  Acc : Outport  Port=2
  Psi : Outport  Port=3
  wires:
  Selector6/1 -> Acc/1
  Kalman Filter/1 -> Selector6/1, Selector5/1, Selector1/1
  In1/1 -> Kalman Filter/1
  Selector5/1 -> Vel/1
  Selector1/1 -> Psi/1

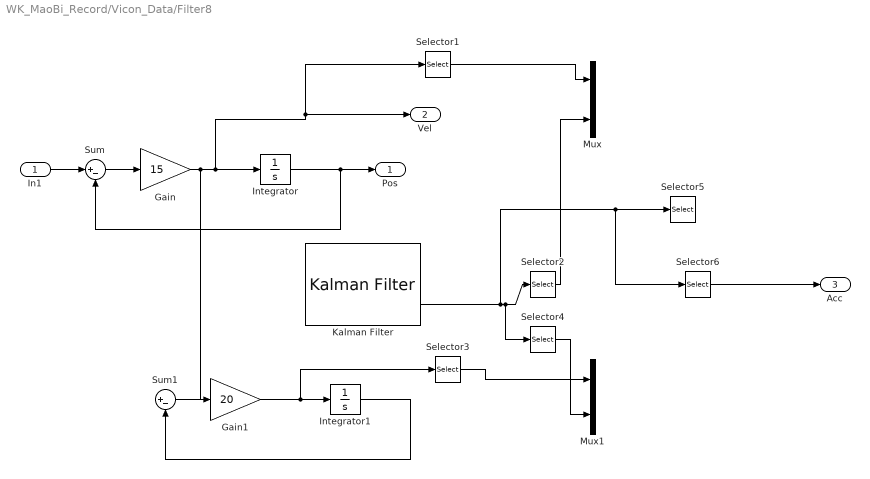
== system WK_MaoBi_Record/Vicon_Data/Filter8 ==
  In1 : Inport
  Gain : Gain  Gain=15
  Gain1 : Gain  Gain=20
  Integrator : Integrator
  Integrator1 : Integrator
  Kalman Filter : dspadpt3/Kalman Filter  SystemSampleTime=-1  num_targets=1  sourceEnable=Always  isReset=on  X=zeros([9, 1])  P=zeros(9)  A=[1 sample_time sample_time*sample_time/2 zeros(1,6);0 1 sample_time zeros(1,6);0 0 1 zeros(1,6);0 0 0 1 sample_time sample_time*sample_time/2 0 0 0;zeros(1,4) 1 sample_time zeros(1,3);zeros(1,5) 1 zeros(1,3);zeros(1,6) 1 sample_time sample_time*sample_time/2;zeros(1,7) 1 sample_time;zeros(1,8) 1]  sourceMeasure=Specify via Dialog  H=[1 zeros(1,8); zeros(1,3) 1 zeros(1,5);zeros(1,6) 1 0 0]  Q=diag([0 0.001 0.001 0 0.001 0.001 0 0.001 0.001])  R=0.001*eye(3)  isOutputEstMeasure=on  isOutputEstState=on  isOutputEstError=off  isOutputPrdMeasure=off  isOutputPrdState=off  isOutputPrdError=off
  Mux : Mux  Inputs=2
  Mux1 : Mux  Inputs=2
  Selector1 : Selector  InputPortWidth=3  IndexOptions=Index vector (dialog)  Indices=[2]  OutputSizes=1
  Selector2 : Selector  InputPortWidth=9  IndexOptions=Index vector (dialog)  Indices=[5]  OutputSizes=1
  Selector3 : Selector  InputPortWidth=3  IndexOptions=Index vector (dialog)  Indices=[2]  OutputSizes=1
  Selector4 : Selector  InputPortWidth=9  IndexOptions=Index vector (dialog)  Indices=[6]  OutputSizes=1
  Selector5 : Selector  InputPortWidth=9  IndexOptions=Index vector (dialog)  Indices=[2 5 8]  OutputSizes=1
  Selector6 : Selector  InputPortWidth=9  IndexOptions=Index vector (dialog)  Indices=[3 6 9]  OutputSizes=1
  Sum : Sum  Inputs=|+-
  Sum1 : Sum  Inputs=|+-
  Pos : Outport
  Vel : Outport  Port=2
  Acc : Outport  Port=3
  wires:
  Sum/1 -> Gain/1
  Gain/1 -> Integrator/1, Selector1/1, Vel/1, Sum1/1
  Integrator/1 -> Pos/1, Sum/2
  In1/1 -> Sum/1
  Selector1/1 -> Mux/1
  Kalman Filter/2 -> Selector4/1, Selector2/1, Selector5/1, Selector6/1
  Sum1/1 -> Gain1/1
  Gain1/1 -> Integrator1/1, Selector3/1
  Integrator1/1 -> Sum1/2
  Selector2/1 -> Mux/2
  Selector3/1 -> Mux1/1
  Selector4/1 -> Mux1/2
  Selector6/1 -> Acc/1

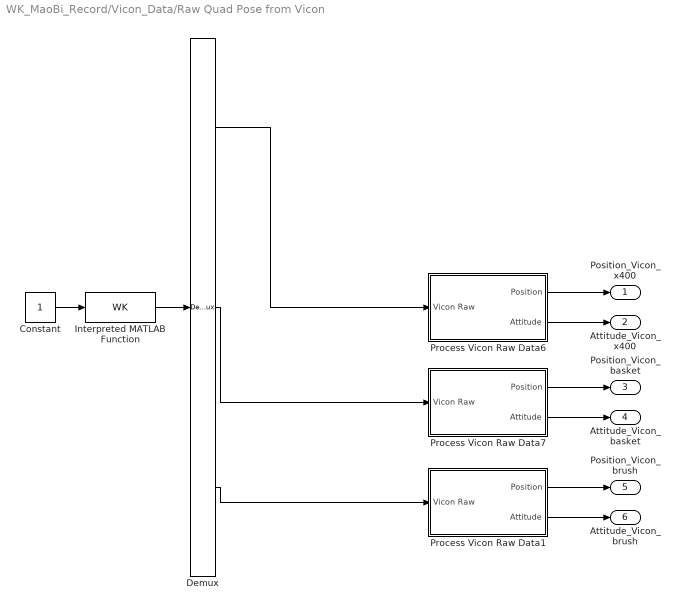
== system WK_MaoBi_Record/Vicon_Data/Raw Quad Pose from Vicon ==
  Constant : Constant
  Demux : Demux  Outputs=3
  Interpreted MATLAB Function : MATLABFcn  MATLABFcn=WK
  Process Vicon Raw Data1 : Subsystem
  Process Vicon Raw Data6 : Subsystem
  Process Vicon Raw Data7 : Subsystem
  Position_Vicon_x400 : Outport
  Attitude_Vicon_x400 : Outport  Port=2
  Position_Vicon_basket : Outport  Port=3
  Attitude_Vicon_basket : Outport  Port=4
  Position_Vicon_brush : Outport  Port=5
  Attitude_Vicon_brush : Outport  Port=6
  wires:
  Interpreted MATLAB Function/1 -> Demux/1
  Process Vicon Raw Data6/2(Attitude) -> Attitude_Vicon_x400/1
  Process Vicon Raw Data6/1(Position) -> Position_Vicon_x400/1
  Demux/1 -> Process Vicon Raw Data6/1(Vicon Raw)
  Constant/1 -> Interpreted MATLAB Function/1
  Process Vicon Raw Data7/2(Attitude) -> Attitude_Vicon_basket/1
  Process Vicon Raw Data7/1(Position) -> Position_Vicon_basket/1
  Demux/2 -> Process Vicon Raw Data7/1(Vicon Raw)
  Process Vicon Raw Data1/2(Attitude) -> Attitude_Vicon_brush/1
  Process Vicon Raw Data1/1(Position) -> Position_Vicon_brush/1
  Demux/3 -> Process Vicon Raw Data1/1(Vicon Raw)

== system WK_MaoBi_Record/Planning/Yaw Controller/Heading ==
  u : Inport  SampleTime=SampleTime
  RESET : Inport  Port=2  SampleTime=SampleTime
  Integral Gain : Gain  DisableCoverage=on  Gain=I  ParamMin=IParamMin  ParamMax=IParamMax  ParamDataTypeStr=IParamDataTypeStr  OutMin=IOutMin  OutMax=IOutMax  OutDataTypeStr=IOutDataTypeStr
  Integrator : DiscreteIntegrator  DisableCoverage=on  IntegratorMethod=Integration: Trapezoidal  ExternalReset=rising  InitialCondition=InitialConditionForIntegrator  InitialConditionMode=State only (most efficient)  SampleTime=-1  OutMin=IntegratorOutMin  OutMax=IntegratorOutMax  OutDataTypeStr=IntegratorOutDataTypeStr  ICPrevOutput=DiscIntNeverNeededParam  ICPrevScaledInput=DiscIntNeverNeededParam
  Proportional Gain : Gain  DisableCoverage=on  Gain=P  ParamMin=PParamMin  ParamMax=PParamMax  ParamDataTypeStr=PParamDataTypeStr  OutMin=POutMin  OutMax=POutMax  OutDataTypeStr=POutDataTypeStr
  Saturation : Saturate  UpperLimit=UpperSaturationLimit  LowerLimit=LowerSaturationLimit  LinearizeAsGain=off  OutMin=SaturationOutMin  OutMax=SaturationOutMax  OutDataTypeStr=SaturationOutDataTypeStr
  Sum : Sum  DisableCoverage=on  Inputs=++|  AccumDataTypeStr=SumAccumDataTypeStr  OutMin=SumOutMin  OutMax=SumOutMax  OutDataTypeStr=SumOutDataTypeStr
  y : Outport  InitialOutput=0
  wires:
  Sum/1 -> Saturation/1
  Saturation/1 -> y/1
  RESET/1 -> Integrator/2
  Proportional Gain/1 -> Sum/1
  Integrator/1 -> Sum/2
  Integral Gain/1 -> Integrator/1
  u/1 -> Proportional Gain/1, Integral Gain/1

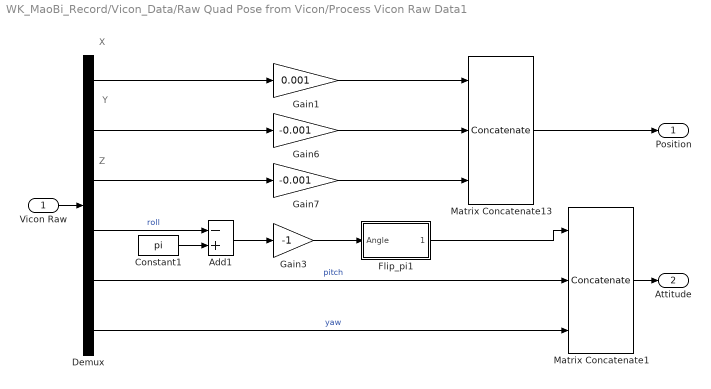
== system WK_MaoBi_Record/Vicon_Data/Raw Quad Pose from Vicon/Process Vicon Raw Data1 ==
  note: X
  note: Y
  note: Z
  Vicon Raw : Inport
  Add1 : Sum  Inputs=-+
  Constant1 : Constant  Value=pi  OutDataTypeStr=double
  Demux : Demux  Outputs=6
  Flip_pi1 : Subsystem
      mask Type: Flip -pi to pi
      mask Description: Flips the inputs into the range -pi to pi
      mask Help: Flips the inputs into the range -pi to pi
      mask Display: disp('Flip_pi')
  Gain1 : Gain  Gain=0.001
  Gain3 : Gain  Gain=-1
  Gain6 : Gain  Gain=-0.001
  Gain7 : Gain  Gain=-0.001
  Matrix Concatenate1 : Concatenate  NumInputs=3  Mode=Multidimensional array
  Matrix Concatenate13 : Concatenate  NumInputs=3  Mode=Multidimensional array
  Position : Outport
  Attitude : Outport  Port=2
  wires:
  Constant1/1 -> Add1/2
  Demux/6 -> Matrix Concatenate1/3  "yaw"
  Gain1/1 -> Matrix Concatenate13/1
  Demux/1 -> Gain1/1
  Demux/2 -> Gain6/1
  Demux/3 -> Gain7/1
  Demux/4 -> Add1/1  "roll"
  Gain6/1 -> Matrix Concatenate13/2
  Gain7/1 -> Matrix Concatenate13/3
  Add1/1 -> Gain3/1
  Gain3/1 -> Flip_pi1/1(Angle)
  Demux/5 -> Matrix Concatenate1/2  "pitch"
  Flip_pi1/1(Angle_Flip) -> Matrix Concatenate1/1
  Matrix Concatenate13/1 -> Position/1
  Vicon Raw/1 -> Demux/1
  Matrix Concatenate1/1 -> Attitude/1

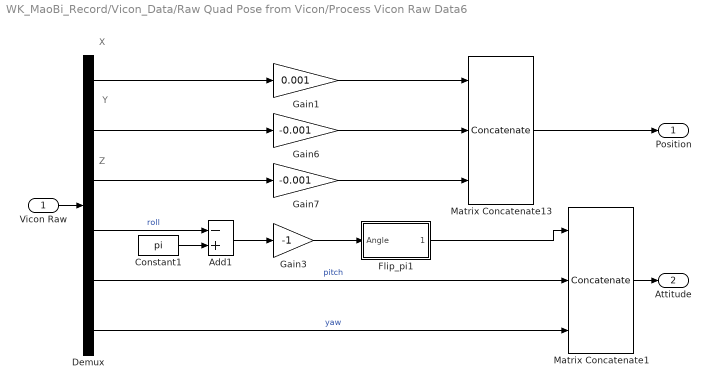
== system WK_MaoBi_Record/Vicon_Data/Raw Quad Pose from Vicon/Process Vicon Raw Data6 ==
  note: X
  note: Y
  note: Z
  Vicon Raw : Inport
  Add1 : Sum  Inputs=-+
  Constant1 : Constant  Value=pi  OutDataTypeStr=double
  Demux : Demux  Outputs=6
  Flip_pi1 : Subsystem
      mask Type: Flip -pi to pi
      mask Description: Flips the inputs into the range -pi to pi
      mask Help: Flips the inputs into the range -pi to pi
      mask Display: disp('Flip_pi')
  Gain1 : Gain  Gain=0.001
  Gain3 : Gain  Gain=-1
  Gain6 : Gain  Gain=-0.001
  Gain7 : Gain  Gain=-0.001
  Matrix Concatenate1 : Concatenate  NumInputs=3  Mode=Multidimensional array
  Matrix Concatenate13 : Concatenate  NumInputs=3  Mode=Multidimensional array
  Position : Outport
  Attitude : Outport  Port=2
  wires:
  Constant1/1 -> Add1/2
  Demux/6 -> Matrix Concatenate1/3  "yaw"
  Gain1/1 -> Matrix Concatenate13/1
  Demux/1 -> Gain1/1
  Demux/2 -> Gain6/1
  Demux/3 -> Gain7/1
  Demux/4 -> Add1/1  "roll"
  Gain6/1 -> Matrix Concatenate13/2
  Gain7/1 -> Matrix Concatenate13/3
  Add1/1 -> Gain3/1
  Gain3/1 -> Flip_pi1/1(Angle)
  Demux/5 -> Matrix Concatenate1/2  "pitch"
  Flip_pi1/1(Angle_Flip) -> Matrix Concatenate1/1
  Matrix Concatenate13/1 -> Position/1
  Vicon Raw/1 -> Demux/1
  Matrix Concatenate1/1 -> Attitude/1

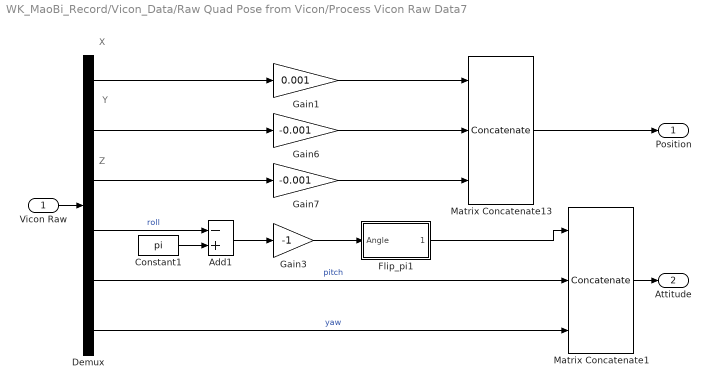
== system WK_MaoBi_Record/Vicon_Data/Raw Quad Pose from Vicon/Process Vicon Raw Data7 ==
  note: Z
  note: Y
  note: X
  Vicon Raw : Inport
  Add1 : Sum  Inputs=-+
  Constant1 : Constant  Value=pi  OutDataTypeStr=double
  Demux : Demux  Outputs=6
  Flip_pi1 : Subsystem
      mask Type: Flip -pi to pi
      mask Description: Flips the inputs into the range -pi to pi
      mask Help: Flips the inputs into the range -pi to pi
      mask Display: disp('Flip_pi')
  Gain1 : Gain  Gain=0.001
  Gain3 : Gain  Gain=-1
  Gain6 : Gain  Gain=-0.001
  Gain7 : Gain  Gain=-0.001
  Matrix Concatenate1 : Concatenate  NumInputs=3  Mode=Multidimensional array
  Matrix Concatenate13 : Concatenate  NumInputs=3  Mode=Multidimensional array
  Position : Outport
  Attitude : Outport  Port=2
  wires:
  Matrix Concatenate1/1 -> Attitude/1
  Vicon Raw/1 -> Demux/1
  Matrix Concatenate13/1 -> Position/1
  Flip_pi1/1(Angle_Flip) -> Matrix Concatenate1/1
  Demux/5 -> Matrix Concatenate1/2  "pitch"
  Gain3/1 -> Flip_pi1/1(Angle)
  Add1/1 -> Gain3/1
  Gain7/1 -> Matrix Concatenate13/3
  Gain6/1 -> Matrix Concatenate13/2
  Demux/4 -> Add1/1  "roll"
  Demux/3 -> Gain7/1
  Demux/2 -> Gain6/1
  Demux/1 -> Gain1/1
  Gain1/1 -> Matrix Concatenate13/1
  Demux/6 -> Matrix Concatenate1/3  "yaw"
  Constant1/1 -> Add1/2

== system WK_MaoBi_Record/Vicon_Data/Raw Quad Pose from Vicon/Process Vicon Raw Data1/Flip_pi1 ==
  Angle : Inport
  Add : Sum  Inputs=-+
  Compare To Constant1 : simulink/Logic and Bit Operations/Compare To Constant  SystemSampleTime=-1  relop=>  const=pi  LogicOutDataTypeMode=uint8  ZeroCross=off
  Constant : Constant  Value=2*pi
  Data Type Duplicate : DataTypeDuplicate
  Flip_0_to_2pi : Subsystem
      mask Type: Flip zero to 2pi
      mask Description: Flips the inputs into the range zero to +2pi
      mask Help: Flips the inputs into the range zero to +2pi
      mask Display: disp('Flip_0_2pi')
  Switch : Switch  Criteria=u2 ~= 0
  Angle_Flip : Outport
  wires:
  Switch/1 -> Data Type Duplicate/1, Angle_Flip/1
  Add/1 -> Switch/1
  Constant/1 -> Add/1
  Compare To Constant1/1 -> Switch/2
  Flip_0_to_2pi/1(Angle_Flip) -> Add/2, Compare To Constant1/1, Switch/3
  Angle/1 -> Data Type Duplicate/2, Flip_0_to_2pi/1(Angle)

== system WK_MaoBi_Record/Vicon_Data/Raw Quad Pose from Vicon/Process Vicon Raw Data6/Flip_pi1 ==
  Angle : Inport
  Add : Sum  Inputs=-+
  Compare To Constant1 : simulink/Logic and Bit Operations/Compare To Constant  SystemSampleTime=-1  relop=>  const=pi  LogicOutDataTypeMode=uint8  ZeroCross=off
  Constant : Constant  Value=2*pi
  Data Type Duplicate : DataTypeDuplicate
  Flip_0_to_2pi : Subsystem
      mask Type: Flip zero to 2pi
      mask Description: Flips the inputs into the range zero to +2pi
      mask Help: Flips the inputs into the range zero to +2pi
      mask Display: disp('Flip_0_2pi')
  Switch : Switch  Criteria=u2 ~= 0
  Angle_Flip : Outport
  wires:
  Switch/1 -> Data Type Duplicate/1, Angle_Flip/1
  Add/1 -> Switch/1
  Constant/1 -> Add/1
  Compare To Constant1/1 -> Switch/2
  Flip_0_to_2pi/1(Angle_Flip) -> Add/2, Compare To Constant1/1, Switch/3
  Angle/1 -> Data Type Duplicate/2, Flip_0_to_2pi/1(Angle)

== system WK_MaoBi_Record/Vicon_Data/Raw Quad Pose from Vicon/Process Vicon Raw Data7/Flip_pi1 ==
  Angle : Inport
  Add : Sum  Inputs=-+
  Compare To Constant1 : simulink/Logic and Bit Operations/Compare To Constant  SystemSampleTime=-1  relop=>  const=pi  LogicOutDataTypeMode=uint8  ZeroCross=off
  Constant : Constant  Value=2*pi
  Data Type Duplicate : DataTypeDuplicate
  Flip_0_to_2pi : Subsystem
      mask Type: Flip zero to 2pi
      mask Description: Flips the inputs into the range zero to +2pi
      mask Help: Flips the inputs into the range zero to +2pi
      mask Display: disp('Flip_0_2pi')
  Switch : Switch  Criteria=u2 ~= 0
  Angle_Flip : Outport
  wires:
  Angle/1 -> Flip_0_to_2pi/1(Angle), Data Type Duplicate/2
  Flip_0_to_2pi/1(Angle_Flip) -> Switch/3, Compare To Constant1/1, Add/2
  Compare To Constant1/1 -> Switch/2
  Constant/1 -> Add/1
  Add/1 -> Switch/1
  Switch/1 -> Angle_Flip/1, Data Type Duplicate/1

== system WK_MaoBi_Record/Vicon_Data/Raw Quad Pose from Vicon/Process Vicon Raw Data1/Flip_pi1/Flip_0_to_2pi ==
  Angle : Inport
  Add : Sum
  Compare To Constant1 : simulink/Logic and Bit Operations/Compare To Constant  SystemSampleTime=-1  relop=<  const=0  LogicOutDataTypeMode=uint8  ZeroCross=off
  Constant : Constant  Value=2*pi
  Data Type Duplicate : DataTypeDuplicate
  Flip_2pi : Subsystem
      mask Type: Flip -2pi to 2pi
      mask Description: Flips the inputs into the range -2pi to +2pi
      mask Help: Flips the inputs into the range -2pi to +2pi
      mask Display: disp('Flip_2pi')
  Switch : Switch  Criteria=u2 ~= 0
  Angle_Flip : Outport
  wires:
  Switch/1 -> Data Type Duplicate/1, Angle_Flip/1
  Angle/1 -> Data Type Duplicate/2, Flip_2pi/1(Angle)
  Add/1 -> Switch/1
  Constant/1 -> Add/1
  Compare To Constant1/1 -> Switch/2
  Flip_2pi/1(Angle_Flip) -> Switch/3, Add/2, Compare To Constant1/1

== system WK_MaoBi_Record/Vicon_Data/Raw Quad Pose from Vicon/Process Vicon Raw Data6/Flip_pi1/Flip_0_to_2pi ==
  Angle : Inport
  Add : Sum
  Compare To Constant1 : simulink/Logic and Bit Operations/Compare To Constant  SystemSampleTime=-1  relop=<  const=0  LogicOutDataTypeMode=uint8  ZeroCross=off
  Constant : Constant  Value=2*pi
  Data Type Duplicate : DataTypeDuplicate
  Flip_2pi : Subsystem
      mask Type: Flip -2pi to 2pi
      mask Description: Flips the inputs into the range -2pi to +2pi
      mask Help: Flips the inputs into the range -2pi to +2pi
      mask Display: disp('Flip_2pi')
  Switch : Switch  Criteria=u2 ~= 0
  Angle_Flip : Outport
  wires:
  Switch/1 -> Data Type Duplicate/1, Angle_Flip/1
  Angle/1 -> Data Type Duplicate/2, Flip_2pi/1(Angle)
  Add/1 -> Switch/1
  Constant/1 -> Add/1
  Compare To Constant1/1 -> Switch/2
  Flip_2pi/1(Angle_Flip) -> Switch/3, Add/2, Compare To Constant1/1

== system WK_MaoBi_Record/Vicon_Data/Raw Quad Pose from Vicon/Process Vicon Raw Data7/Flip_pi1/Flip_0_to_2pi ==
  Angle : Inport
  Add : Sum
  Compare To Constant1 : simulink/Logic and Bit Operations/Compare To Constant  SystemSampleTime=-1  relop=<  const=0  LogicOutDataTypeMode=uint8  ZeroCross=off
  Constant : Constant  Value=2*pi
  Data Type Duplicate : DataTypeDuplicate
  Flip_2pi : Subsystem
      mask Type: Flip -2pi to 2pi
      mask Description: Flips the inputs into the range -2pi to +2pi
      mask Help: Flips the inputs into the range -2pi to +2pi
      mask Display: disp('Flip_2pi')
  Switch : Switch  Criteria=u2 ~= 0
  Angle_Flip : Outport
  wires:
  Flip_2pi/1(Angle_Flip) -> Compare To Constant1/1, Add/2, Switch/3
  Compare To Constant1/1 -> Switch/2
  Constant/1 -> Add/1
  Add/1 -> Switch/1
  Angle/1 -> Flip_2pi/1(Angle), Data Type Duplicate/2
  Switch/1 -> Angle_Flip/1, Data Type Duplicate/1

== system WK_MaoBi_Record/Vicon_Data/Raw Quad Pose from Vicon/Process Vicon Raw Data1/Flip_pi1/Flip_0_to_2pi/Flip_2pi ==
  Angle : Inport
  Bias : Bias  Bias=-2*pi
  Constant : Constant  Value=2*pi
  Data Type Duplicate : DataTypeDuplicate
  Modulo : Math  Operator=mod  SaturateOnIntegerOverflow=on
  Sign1 : Signum
  Switch : Switch
  Angle_Flip : Outport
  wires:
  Switch/1 -> Data Type Duplicate/2, Angle_Flip/1
  Bias/1 -> Switch/3
  Sign1/1 -> Switch/2
  Modulo/1 -> Switch/1, Bias/1
  Constant/1 -> Modulo/2
  Angle/1 -> Data Type Duplicate/1, Sign1/1, Modulo/1

== system WK_MaoBi_Record/Vicon_Data/Raw Quad Pose from Vicon/Process Vicon Raw Data6/Flip_pi1/Flip_0_to_2pi/Flip_2pi ==
  Angle : Inport
  Bias : Bias  Bias=-2*pi
  Constant : Constant  Value=2*pi
  Data Type Duplicate : DataTypeDuplicate
  Modulo : Math  Operator=mod  SaturateOnIntegerOverflow=on
  Sign1 : Signum
  Switch : Switch
  Angle_Flip : Outport
  wires:
  Switch/1 -> Data Type Duplicate/2, Angle_Flip/1
  Bias/1 -> Switch/3
  Sign1/1 -> Switch/2
  Modulo/1 -> Switch/1, Bias/1
  Constant/1 -> Modulo/2
  Angle/1 -> Data Type Duplicate/1, Sign1/1, Modulo/1

== system WK_MaoBi_Record/Vicon_Data/Raw Quad Pose from Vicon/Process Vicon Raw Data7/Flip_pi1/Flip_0_to_2pi/Flip_2pi ==
  Angle : Inport
  Bias : Bias  Bias=-2*pi
  Constant : Constant  Value=2*pi
  Data Type Duplicate : DataTypeDuplicate
  Modulo : Math  Operator=mod  SaturateOnIntegerOverflow=on
  Sign1 : Signum
  Switch : Switch
  Angle_Flip : Outport
  wires:
  Angle/1 -> Modulo/1, Sign1/1, Data Type Duplicate/1
  Constant/1 -> Modulo/2
  Modulo/1 -> Bias/1, Switch/1
  Sign1/1 -> Switch/2
  Bias/1 -> Switch/3
  Switch/1 -> Angle_Flip/1, Data Type Duplicate/2

== matlab function Planning/Yaw Controller/MATLAB Function ==
  data: u input double; y output double
function y = fcn(u)
%#codegen
y = u;
if y > pi    
    y = y - 2*pi;
elseif y < -pi
        y = y + 2*pi;
end
